simulink model "OneCombinedLQR2"  (R2024b)
settings: Solver=ode4  StartTime=0.0  StopTime=T_end  FixedStep=0.005  RelTol=1e-3
values from neighbouring files (symbols this model uses):
  h_ref = double(h_ref)    [main.m]
  K_lqr = double(K_lqr)    [main.m]
  P = [x_ref y_ref]    [main.m]
  S_path = [S_path; S_raw(end)]    [main.m]
  theta_ref_unwrapped = unwrap(theta_ref)    [main.m]
  vd_path = min(vd_path, vd_max)    [main.m]
  wd_path = max(min(wd_path, wd_max), -wd_max)    [main.m]
  x_init = [phi_h; 0; theta_h; 0; v_h; omega_h; x_h; y_h]    [main.m]
settings Model: Creator=mwali  LastModifiedBy=mwali
settings ConfigComp: CovBoundaryAbsTol=1.0e-5

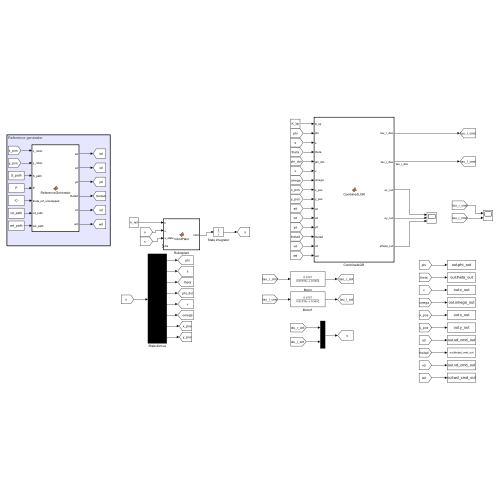
[thumbnail: Simulink's stored preview of the top-level diagram]
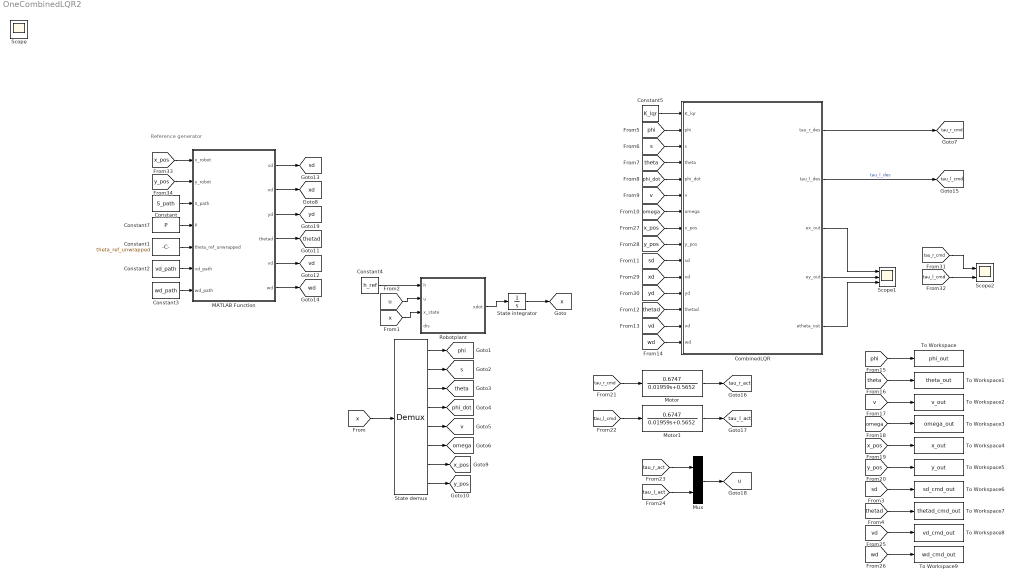
== system OneCombinedLQR2 ==
  note: Reference generator
  CombinedLQR : MATLAB Function  TreatAsAtomicUnit=on
  Constant : Constant  Value=S_path
  Constant1 : Constant  Value=theta_ref_unwrapped
  Constant2 : Constant  Value=vd_path
  Constant3 : Constant  Value=wd_path
  Constant4 : Constant  Value=h_ref
  Constant5 : Constant  Value=K_lqr
  Constant7 : Constant  Value=P
  MATLAB Function : MATLAB Function  TreatAsAtomicUnit=on
  Motor : TransferFcn  Numerator=[0.6747]  Denominator=[0.01959 0.5652]
  Motor1 : TransferFcn  Numerator=[0.6747]  Denominator=[0.01959 0.5652]
  Mux : Mux  Inputs=2
  Robotplant : MATLAB Function  TreatAsAtomicUnit=on
  Scope1 : Scope  NumInputPorts=3
  Scope2 : Scope  NumInputPorts=2
  State demux : Demux  Outputs=8
  State integrator : Integrator  InitialCondition=x_init
  To Workspace : ToWorkspace  VariableName=phi_out  SampleTime=-1
  To Workspace1 : ToWorkspace  VariableName=theta_out  SampleTime=-1
  To Workspace2 : ToWorkspace  VariableName=v_out  SampleTime=-1
  To Workspace3 : ToWorkspace  VariableName=omega_out  SampleTime=-1
  To Workspace4 : ToWorkspace  VariableName=x_out  SampleTime=-1
  To Workspace5 : ToWorkspace  VariableName=y_out  SampleTime=-1
  To Workspace6 : ToWorkspace  VariableName=sd_cmd_out  SampleTime=-1
  To Workspace7 : ToWorkspace  VariableName=thetad_cmd_out  SampleTime=-1
  To Workspace8 : ToWorkspace  VariableName=vd_cmd_out  SampleTime=-1
  To Workspace9 : ToWorkspace  VariableName=wd_cmd_out  SampleTime=-1
  Scope : Scope
  tag scope: omega=global, phi=global, phi_dot=global, s=global, sd=global, tau_l_act=global, tau_l_cmd=global, tau_r_act=global, tau_r_cmd=global, theta=global, thetad=global, u=global, v=global, vd=global, wd=global, x=global, x_pos=global, xd=global, y_pos=global, yd=global
  wires:
  [phi_dot] -> CombinedLQR/5(phi_dot)
  CombinedLQR/2(tau_l_des) -> [tau_l_cmd]  "tau_l_des"
  [thetad] -> CombinedLQR/13(thetad)
  [v] -> CombinedLQR/6(v)
  State integrator/1 -> [x]
  [x] -> State demux/1
  [tau_l_act] -> Mux/2
  [tau_r_cmd] -> Motor/1
  State demux/6 -> [omega]
  [sd] -> CombinedLQR/10(sd)
  Robotplant/1(xdot) -> State integrator/1
  [y_pos] -> To Workspace5/1
  Motor1/1 -> [tau_l_act]
  MATLAB Function/1(sd) -> [sd]
  MATLAB Function/5(vd) -> [vd]
  MATLAB Function/6(wd) -> [wd]
  Constant5/1 -> CombinedLQR/1(K_lqr)
  [wd] -> CombinedLQR/15(wd)
  [theta] -> To Workspace1/1
  Mux/1 -> [u]
  State demux/7 -> [x_pos]
  State demux/2 -> [s]
  [omega] -> To Workspace3/1
  [s] -> CombinedLQR/3(s)
  State demux/1 -> [phi]
  [phi] -> To Workspace/1
  [phi] -> CombinedLQR/2(phi)
  [tau_r_act] -> Mux/1
  State demux/8 -> [y_pos]
  State demux/4 -> [phi_dot]
  [v] -> To Workspace2/1
  [omega] -> CombinedLQR/7(omega)
  [vd] -> CombinedLQR/14(vd)
  Motor/1 -> [tau_r_act]
  State demux/5 -> [v]
  MATLAB Function/4(thetad) -> [thetad]
  [x_pos] -> To Workspace4/1
  State demux/3 -> [theta]
  [tau_l_cmd] -> Motor1/1
  [theta] -> CombinedLQR/4(theta)
  [vd] -> To Workspace8/1
  [wd] -> To Workspace9/1
  [thetad] -> To Workspace7/1
  [sd] -> To Workspace6/1
  MATLAB Function/2(xd) -> [xd]
  MATLAB Function/3(yd) -> [yd]
  [x_pos] -> CombinedLQR/8(x_pos)
  [y_pos] -> CombinedLQR/9(y_pos)
  [xd] -> CombinedLQR/11(xd)
  [yd] -> CombinedLQR/12(yd)
  [tau_r_cmd] -> Scope2/1
  [tau_l_cmd] -> Scope2/2
  Constant1/1 -> MATLAB Function/5(theta_ref_unwrapped)
  Constant7/1 -> MATLAB Function/4(P)
  [x_pos] -> MATLAB Function/1(x_robot)
  [y_pos] -> MATLAB Function/2(y_robot)
  Constant/1 -> MATLAB Function/3(S_path)
  Constant2/1 -> MATLAB Function/6(vd_path)
  Constant3/1 -> MATLAB Function/7(wd_path)
  CombinedLQR/1(tau_r_des) -> [tau_r_cmd]
  [x] -> Robotplant/3(x_state)
  [u] -> Robotplant/2(u)
  Constant4/1 -> Robotplant/1(h)
  CombinedLQR/4(ey_out) -> Scope1/2
  CombinedLQR/3(ex_out) -> Scope1/1
  CombinedLQR/5(etheta_out) -> Scope1/3

== matlab function OneCombinedLQR2/CombinedLQR ==
  settings: updateMethod=DISCRETE
  data: K_lqr input; phi input; s input; theta input; phi_dot input; v input; omega input; x_pos input; y_pos input; sd input; xd input; yd input; thetad input; vd input; wd input; tau_r_des output; tau_l_des output; ex_out output; ey_out output; etheta_out output
function [tau_r_des, tau_l_des, ex_out, ey_out, etheta_out] = CombinedLQR( ...
    K_lqr, phi, s, theta, phi_dot, v, omega, x_pos, y_pos, ...
    sd, xd, yd, thetad, vd, wd)
%#codegen

% outputs init
tau_r_des  = 0;
tau_l_des  = 0;
ex_out     = 0;
ey_out     = 0;
etheta_out = 0;

% -----------------------------
% 1) Path position error in world frame
% -----------------------------
dx = xd - x_pos;
dy = yd - y_pos;

% -----------------------------
% 2) Error in robot body frame
% ex = forward error
% et = lateral error
% -----------------------------
ex =  cos(theta)*dx + sin(theta)*dy;
ey = -sin(theta)*dx + cos(theta)*dy;

% save for plotting
ex_out = ex;
ey_out = ey;

% -----------------------------
% 3) Heading correction from lateral error
% -----------------------------
k_y = 0.1;                     % tune this if needed
theta_corr_max = deg2rad(20);  % max heading correction

theta_corr = k_y * ey;

if theta_corr > theta_corr_max
    theta_corr = theta_corr_max;
elseif theta_corr < -theta_corr_max
    theta_corr = -theta_corr_max;
end

thetad_corr = thetad + theta_corr;

% -----------------------------
% 4) State error for LQR
% -----------------------------
e = zeros(6,1);
e(1) =phi ;
e(2) = s - sd; 
e(3) = atan2(sin(theta - thetad_corr), cos(theta - thetad_corr));
e(4) = phi_dot;
e(5) = v - vd;
e(6) = omega - wd;

etheta_out = e(3);

% -----------------------------
% 5) LQR control
% -----------------------------
u_des = -K_lqr * e;

tau_r_des = u_des(1);
tau_l_des = u_des(2);

% -----------------------------
% 6) Torque saturation
% -----------------------------
tau_lim = 50; % Changed from 6 to 3

if tau_r_des > tau_lim
    tau_r_des = tau_lim;
elseif tau_r_des < -tau_lim
    tau_r_des = -tau_lim;
end

if tau_l_des > tau_lim
    tau_l_des = tau_lim;
elseif tau_l_des < -tau_lim
    tau_l_des = -tau_lim;
end

== matlab function OneCombinedLQR2/MATLAB Function ==
  data: x_robot input; y_robot input; S_path input; P input; theta_ref_unwrapped input; vd_path input; wd_path input; sd output; xd output; yd output; thetad output; vd output; wd output
function [sd, xd, yd, thetad, vd, wd] = ReferenceGenerator(x_robot, y_robot, S_path, P, theta_ref_unwrapped, vd_path, wd_path)
    N = size(P, 1);

    % 1. Find the nearest discrete node
    min_dist2 = inf;
    k_min = int32(1);
    for k = int32(1) : int32(N)
        dx = P(k, 1) - x_robot;
        dy = P(k, 2) - y_robot;
        d2 = dx*dx + dy*dy;
        if d2 < min_dist2
            min_dist2 = d2;
            k_min = k;
        end
    end

    % 2. Continuous Projection (Fixes the high-frequency torque chattering)
    k_next = min(k_min + int32(1), int32(N));
    k_prev = max(k_min - int32(1), int32(1));

    d2_next = (P(k_next,1)-x_robot)^2 + (P(k_next,2)-y_robot)^2;
    d2_prev = (P(k_prev,1)-x_robot)^2 + (P(k_prev,2)-y_robot)^2;

    if d2_next < d2_prev
        k1 = k_min;
        k2 = k_next;
    else
        k1 = k_prev;
        k2 = k_min;
    end

    if k1 == k2
        alpha = 0.0;
    else
        vx = P(k2,1) - P(k1,1);
        vy = P(k2,2) - P(k1,2);
        L2 = vx*vx + vy*vy;
        if L2 > 1e-6
            rx = x_robot - P(k1,1);
            ry = y_robot - P(k1,2);
            % Orthogonal projection scalar
            alpha = (rx*vx + ry*vy) / L2;
            alpha = max(0.0, min(1.0, alpha));
        else
            alpha = 0.0;
        end
    end

    % 3. Interpolate perfectly smooth references (No Lookahead)
    sd     = (1 - alpha) * S_path(k1) + alpha * S_path(k2);
    xd     = (1 - alpha) * P(k1, 1)   + alpha * P(k2, 1);
    yd     = (1 - alpha) * P(k1, 2)   + alpha * P(k2, 2);
    thetad = (1 - alpha) * theta_ref_unwrapped(k1) + alpha * theta_ref_unwrapped(k2);
    vd     = (1 - alpha) * vd_path(k1) + alpha * vd_path(k2);
    wd     = (1 - alpha) * wd_path(k1) + alpha * wd_path(k2);

    % 4. Safety clamps
    vd_max = 0.3;
    wd_max = 0.334;
    vd = max(0, min(vd, vd_max));
    wd = max(min(wd, wd_max), -wd_max);
end

== matlab function OneCombinedLQR2/Robotplant ==
  data: h input; u input; xdot output; x_state input; dis input
function xdot = robotPlant(h, u, x_state,dis)

xdot = zeros(8,1);

% ---- Physical constants ----
Mw = 0.150;
Mb = 11.3;
r  = 0.060;
d  = 0.450;
Iw = 0.0002757224;
g  = 9.81;

% ---- Height-dependent parameters ----
Lc = -0.4748*h^2 + 1.2434*h - 0.0286;   % CoM height above wheel axle
Iy =  1.4948*h^2 + 0.5774*h - 0.0053;
Iz = -0.5689*h^2 + 0.1583*h + 0.1236;

% ---- Inertia matrix entries ----
M11   = Mb*Lc^2 + Iy;
M12   = Mb*Lc;
M22   = Mb + 2*Mw + 2*Iw/r^2;
M33   = (d^2/2)*Mw + (d^2/(2*r^2))*Iw + Iz;
Delta = M11*M22 - M12^2;

% Numerical safety
if abs(Delta) < 1e-8;  Delta = sign(Delta+1e-10)*1e-8; end
if abs(M33)   < 1e-8;  M33   = 1e-8; end

% ---- Unpack state ----
phi     = x_state(1);
% s     = x_state(2);   % not needed for dynamics
% theta = x_state(3);   % not needed for dynamics
phi_dot = x_state(4);
v       = x_state(5);
% omega = x_state(6);   % not needed for dynamics
theta_now = x_state(3);

% ---- Control inputs ----
tau_r = u(1);   % right-wheel torque [N*m]
tau_l = u(2);   % left-wheel torque  [N*m]

tau_sum  = tau_r + tau_l;
tau_diff = tau_r - tau_l;

% ---- Nonlinear generalized forces ----
% (derived from Lagrangian; see e.g. Grasser et al. 2002)
F_phi  = -M12 / (r * Delta) * tau_sum;           % torque -> phi_ddot channel
F_v    =  M11 / (r * Delta) * tau_sum;           % torque -> v_dot channel
F_yaw  =  d   / (2 * r * M33) * tau_diff;        % torque -> omega_dot channel

gravity_phi = (M22 * Mb * g * Lc) / Delta;       % phi channel gravity term
gravity_v   = (-M12 * Mb * g * Lc) / Delta;      % v channel gravity term
C_air = 2.5; 
wind_disturbance = -C_air * v * abs(v); 

% ---- FIX #1: nonlinear gravity term uses sin(phi) not phi ---- 
% Add the wind_disturbance to the pitch dynamics
phi_ddot  = gravity_phi * sin(phi) + F_phi + wind_disturbance + dis;
v_dot     = gravity_v   * sin(phi) + F_v;
omega_dot = F_yaw;

% ---- Kinematics ----
x_pos_dot = v * cos(theta_now);
y_pos_dot = v * sin(theta_now);

% ---- Assemble xdot ----
% [phi; s; theta; phi_dot; v; omega; x_pos; y_pos]
xdot(1) = phi_dot;        % d(phi)/dt
xdot(2) = v;              % d(s)/dt   = forward speed
xdot(3) = x_state(6);    % d(theta)/dt = omega
xdot(4) = phi_ddot;       % d(phi_dot)/dt  -- FIX #1
xdot(5) = v_dot;          % d(v)/dt        -- FIX #1
xdot(6) = omega_dot;      % d(omega)/dt
xdot(7) = x_pos_dot;      % d(x_pos)/dt
xdot(8) = y_pos_dot;      % d(y_pos)/dt
